simulink model "multi_level_inverter"  (Simulink 7.3)
settings: Solver=ode3  StartTime=0.0  StopTime=10  FixedStep=1e-4  RelTol=1e-3
libraries: powerlib x61, simulink x4
settings Model: Creator=Administrator  LastModifiedBy=AbdullahBaig
settings OptimizationCC: InitFltsAndDblsToZero=on
settings DebuggingCC: SaveWithParameterizedLinksMsg=none
settings RTWCC: IncludeERTFirstTime=on

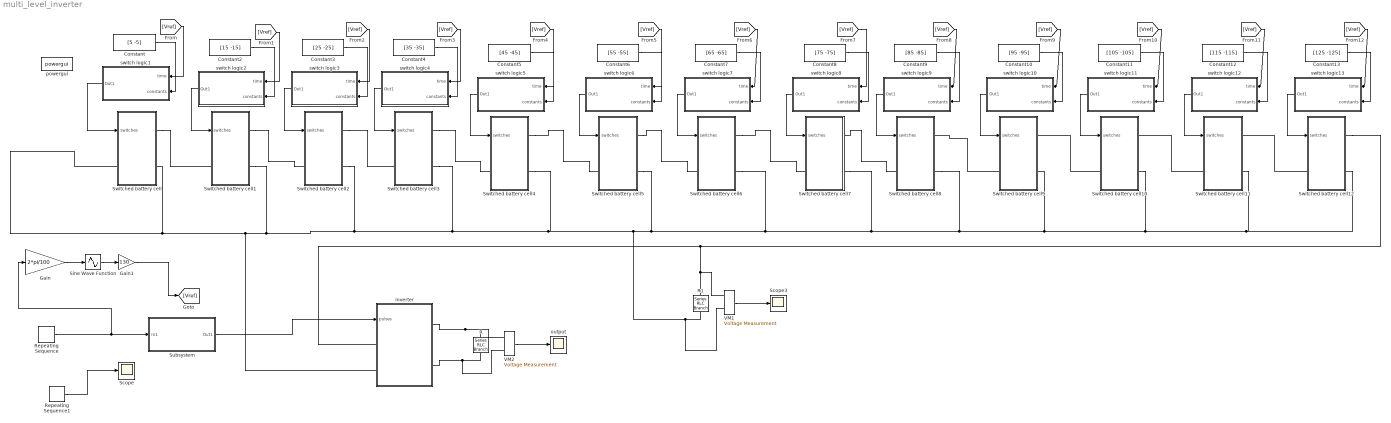
== system multi_level_inverter ==
  Constant : Constant  Value=[5 -5]  OutDataType=fixdt(1, 16)  OutScaling=2^0
  Constant10 : Constant  Value=[95 -95]  OutDataType=fixdt(1, 16)  OutScaling=2^0
  Constant11 : Constant  Value=[105 -105]  OutDataType=fixdt(1, 16)  OutScaling=2^0
  Constant12 : Constant  Value=[115 -115]  OutDataType=fixdt(1, 16)  OutScaling=2^0
  Constant13 : Constant  Value=[125 -125]  OutDataType=fixdt(1, 16)  OutScaling=2^0
  Constant2 : Constant  Value=[15 -15]  OutDataType=fixdt(1, 16)  OutScaling=2^0
  Constant3 : Constant  Value=[25 -25]  OutDataType=fixdt(1, 16)  OutScaling=2^0
  Constant4 : Constant  Value=[35 -35]  OutDataType=fixdt(1, 16)  OutScaling=2^0
  Constant5 : Constant  Value=[45 -45]  OutDataType=fixdt(1, 16)  OutScaling=2^0
  Constant6 : Constant  Value=[55 -55]  OutDataType=fixdt(1, 16)  OutScaling=2^0
  Constant7 : Constant  Value=[65 -65]  OutDataType=fixdt(1, 16)  OutScaling=2^0
  Constant8 : Constant  Value=[75 -75]  OutDataType=fixdt(1, 16)  OutScaling=2^0
  Constant9 : Constant  Value=[85 -85]  OutDataType=fixdt(1, 16)  OutScaling=2^0
  Gain : Gain  Gain=2*pi/100  ParameterDataType=fixdt(1, 16)  ParameterScaling=2^0  OutDataType=fixdt(1, 16)  OutScaling=2^0
  Gain1 : Gain  Gain=130  ParameterDataType=fixdt(1, 16)  ParameterScaling=2^0  OutDataType=fixdt(1, 16)  OutScaling=2^0
  R : powerlib/Elements/Series RLC Branch  DialogController=POWERSYS.PowerSysDialog  PhysicalDomain=powersysdomain  SubClassName=unknown  LeftPortType=p1  RightPortType=p1  LConnTagsString=__new0  RConnTagsString=__new0  BranchType=R  Resistance=500  Inductance=1.0  SetiL0=off  InitialCurrent=0  Capacitance=1.0  Setx0=off  InitialVoltage=0  Measurements=None
  R1 : powerlib/Elements/Series RLC Branch  DialogController=POWERSYS.PowerSysDialog  PhysicalDomain=powersysdomain  SubClassName=unknown  LeftPortType=p1  RightPortType=p1  LConnTagsString=__new0  RConnTagsString=__new0  BranchType=R  Resistance=500  Inductance=1.0  SetiL0=off  InitialCurrent=0  Capacitance=1.0  Setx0=off  InitialVoltage=0  Measurements=None
  Repeating Sequence : simulink/Sources/Repeating Sequence  SystemSampleTime=-1  rep_seq_t=[0 0.02]  rep_seq_y=[0 100]
  Repeating Sequence1 : simulink/Sources/Repeating Sequence  SystemSampleTime=-1  rep_seq_t=[0 0.02]  rep_seq_y=[0 100]
  Scope : Scope
      settings: SaveName=ScopeData2
  Scope3 : Scope
      settings: YMin=0  YMax=250
  Sine Wave Function : Sin  TimeSource=Use external signal  Amplitude=1  Bias=0  Frequency=1  Phase=0  Samples=10  SampleTime=0  Offset=0
  Subsystem : Subsystem
  Switched battery cell : Subsystem
  Switched battery cell1 : Subsystem
  Switched battery cell10 : Subsystem
  Switched battery cell11 : Subsystem
  Switched battery cell12 : Subsystem
  Switched battery cell2 : Subsystem
  Switched battery cell3 : Subsystem
  Switched battery cell4 : Subsystem
  Switched battery cell5 : Subsystem
  Switched battery cell6 : Subsystem
  Switched battery cell7 : Subsystem
  Switched battery cell8 : Subsystem
  Switched battery cell9 : Subsystem
  VM1 : powerlib/Measurements/Voltage Measurement  Tag=PoWeRsYsTeMmEaSuReMeNt  DialogController=POWERSYS.PowerSysDialog  SystemSampleTime=-1  PhasorSimulation=off  OutputType=Magnitude  PSBequivalent=0
  VM2 : powerlib/Measurements/Voltage Measurement  Tag=PoWeRsYsTeMmEaSuReMeNt  DialogController=POWERSYS.PowerSysDialog  SystemSampleTime=-1  PhasorSimulation=off  OutputType=Magnitude  PSBequivalent=0
  inverter : Subsystem
  output : Scope
      settings: YMin=-350  YMax=350
  powergui : powerlib/powergui  SystemSampleTime=-1  SimulationMode=Continuous  SampleTime=50e-6  frequency=60  SPID=off  DisableSnubberDevices=off  DisableRonSwitches=off  DisableVfSwitches=off  SwTol=0  Interpol=off  frequencyindice=0  echomessages=off  HookPort=off  DisplayEquations=off  FunctionMessages=off  EnableUseOfTLC=off  x0status=blocks  RestoreLinks=warning  Frange=[0:2:500]  Ylog=off  Xlog=on  ShowGrid=off  save=off  variable=ZData  ZoomFFT=on  StartTime=0.0  cycles=1  DisplayStyle=1  fundamental=60  FreqAxis=off  MaxFrequency=1000  frequencyindicesteady=1  RmsSteady=1  display=off  Ts=0  methode=off
  switch logic1 : Subsystem
  switch logic10 : Subsystem
  switch logic11 : Subsystem
  switch logic12 : Subsystem
  switch logic13 : Subsystem
  switch logic2 : Subsystem
  switch logic3 : Subsystem
  switch logic4 : Subsystem
  switch logic5 : Subsystem
  switch logic6 : Subsystem
  switch logic7 : Subsystem
  switch logic8 : Subsystem
  switch logic9 : Subsystem
  wires:
  Subsystem/1(Out1) -> inverter/1(pulses)
  VM2/1 -> output/1
  Constant/1 -> switch logic1/2(constants)
  switch logic1/1(Out1) -> Switched battery cell/1(switches)
  Gain/1 -> Sine Wave Function/1
  Sine Wave Function/1 -> Gain1/1
  switch logic2/1(Out1) -> Switched battery cell1/1(switches)
  switch logic3/1(Out1) -> Switched battery cell2/1(switches)
  switch logic4/1(Out1) -> Switched battery cell3/1(switches)
  switch logic5/1(Out1) -> Switched battery cell4/1(switches)
  Constant2/1 -> switch logic2/2(constants)
  Constant3/1 -> switch logic3/2(constants)
  Constant4/1 -> switch logic4/2(constants)
  Constant5/1 -> switch logic5/2(constants)
  switch logic6/1(Out1) -> Switched battery cell5/1(switches)
  Constant6/1 -> switch logic6/2(constants)
  switch logic7/1(Out1) -> Switched battery cell6/1(switches)
  Constant7/1 -> switch logic7/2(constants)
  switch logic8/1(Out1) -> Switched battery cell7/1(switches)
  Constant8/1 -> switch logic8/2(constants)
  switch logic9/1(Out1) -> Switched battery cell8/1(switches)
  Constant9/1 -> switch logic9/2(constants)
  Gain1/1 -> [Vref]
  [Vref] -> switch logic1/1(time)
  [Vref] -> switch logic2/1(time)
  [Vref] -> switch logic3/1(time)
  [Vref] -> switch logic4/1(time)
  [Vref] -> switch logic5/1(time)
  [Vref] -> switch logic6/1(time)
  [Vref] -> switch logic7/1(time)
  [Vref] -> switch logic8/1(time)
  [Vref] -> switch logic9/1(time)
  switch logic10/1(Out1) -> Switched battery cell9/1(switches)
  Constant10/1 -> switch logic10/2(constants)
  [Vref] -> switch logic10/1(time)
  switch logic11/1(Out1) -> Switched battery cell10/1(switches)
  Constant11/1 -> switch logic11/2(constants)
  [Vref] -> switch logic11/1(time)
  switch logic12/1(Out1) -> Switched battery cell11/1(switches)
  Constant12/1 -> switch logic12/2(constants)
  [Vref] -> switch logic12/1(time)
  switch logic13/1(Out1) -> Switched battery cell12/1(switches)
  Constant13/1 -> switch logic13/2(constants)
  [Vref] -> switch logic13/1(time)
  Repeating Sequence/1 -> Subsystem/1(In1), Gain/1
  VM1/1 -> Scope3/1
  Repeating Sequence1/1 -> Scope/1
  connections:
  inverter/RConn1 -- R/LConn1 -- VM2/LConn1
  R/RConn1 -- inverter/RConn2 -- VM2/LConn2
  R1/RConn1 -- Switched battery cell5/RConn2 -- Switched battery cell6/RConn2 -- Switched battery cell7/RConn2 -- Switched battery cell8/RConn2 -- Switched battery cell9/RConn2 -- Switched battery cell10/RConn2 -- Switched battery cell11/RConn2 -- Switched battery cell12/RConn2 -- Switched battery cell/LConn1 -- Switched battery cell/RConn2 -- inverter/LConn2 -- Switched battery cell1/RConn2 -- Switched battery cell2/RConn2 -- Switched battery cell3/RConn2 -- Switched battery cell4/RConn2 -- VM1/LConn2
  Switched battery cell1/RConn1 -- Switched battery cell2/LConn1
  Switched battery cell2/RConn1 -- Switched battery cell3/LConn1
  Switched battery cell3/RConn1 -- Switched battery cell4/LConn1
  Switched battery cell/RConn1 -- Switched battery cell1/LConn1
  Switched battery cell4/RConn1 -- Switched battery cell5/LConn1
  Switched battery cell5/RConn1 -- Switched battery cell6/LConn1
  Switched battery cell6/RConn1 -- Switched battery cell7/LConn1
  Switched battery cell7/RConn1 -- Switched battery cell8/LConn1
  Switched battery cell12/RConn1 -- inverter/LConn1 -- R1/LConn1 -- VM1/LConn1
  Switched battery cell10/LConn1 -- Switched battery cell9/RConn1
  Switched battery cell11/LConn1 -- Switched battery cell10/RConn1
  Switched battery cell12/LConn1 -- Switched battery cell11/RConn1
  Switched battery cell9/LConn1 -- Switched battery cell8/RConn1

== system multi_level_inverter/Subsystem ==
  In1 : Inport
  Compare To Constant : simulink/Logic and Bit Operations/Compare To Constant  SystemSampleTime=-1  relop=>  const=51  LogicOutDataTypeMode=uint8  ZeroCross=off
  Compare To Constant1 : simulink/Logic and Bit Operations/Compare To Constant  SystemSampleTime=-1  relop=<  const=49  LogicOutDataTypeMode=uint8  ZeroCross=off
  Mux : Mux
  Out1 : Outport
  wires:
  Compare To Constant/1 -> Mux/1, Mux/4
  In1/1 -> Compare To Constant/1, Compare To Constant1/1
  Mux/1 -> Out1/1
  Compare To Constant1/1 -> Mux/2, Mux/3

== system multi_level_inverter/Switched battery cell ==
  switches : Inport  OutDataType=fixdt(1, 16)  OutScaling=2^0
  DC Voltage Source : powerlib/Electrical Sources/DC Voltage Source  DialogController=POWERSYS.PowerSysDialog  SystemSampleTime=-1  Amplitude=24  Measurements=None
  Demux : Demux  Outputs=3
  Ideal Switch : powerlib/Power Electronics/Ideal Switch  DialogController=POWERSYS.PowerSysDialog  SystemSampleTime=-1  Ron=0.1  Lon=0  IC=0  Rs=1e5  Cs=inf  Measurements=on
  Ideal Switch1 : powerlib/Power Electronics/Ideal Switch  DialogController=POWERSYS.PowerSysDialog  SystemSampleTime=-1  Ron=0.1  Lon=0  IC=0  Rs=1e5  Cs=inf  Measurements=on
  Ideal Switch2 : powerlib/Power Electronics/Ideal Switch  DialogController=POWERSYS.PowerSysDialog  SystemSampleTime=-1  Ron=0.1  Lon=0  IC=0  Rs=1e5  Cs=inf  Measurements=on
  Conn1 : PMIOPort  Port=1  Side=Right
  Conn2 : PMIOPort  Port=2  Side=Left
  Conn4 : PMIOPort  Port=3  Side=Right
  wires:
  Demux/1 -> Ideal Switch1/1
  Demux/2 -> Ideal Switch2/1
  Demux/3 -> Ideal Switch/1
  switches/1 -> Demux/1
  connections:
  Ideal Switch1/LConn1 -- Ideal Switch2/RConn1 -- Conn2/RConn1
  DC Voltage Source/LConn1 -- Ideal Switch2/LConn1 -- Ideal Switch/RConn1
  DC Voltage Source/RConn1 -- Conn1/RConn1 -- Ideal Switch1/RConn1
  Conn4/RConn1 -- Ideal Switch/LConn1

== system multi_level_inverter/Switched battery cell1 ==
  switches : Inport  OutDataType=fixdt(1, 16)  OutScaling=2^0
  DC Voltage Source : powerlib/Electrical Sources/DC Voltage Source  DialogController=POWERSYS.PowerSysDialog  SystemSampleTime=-1  Amplitude=24  Measurements=None
  Demux : Demux  Outputs=3
  Ideal Switch : powerlib/Power Electronics/Ideal Switch  DialogController=POWERSYS.PowerSysDialog  SystemSampleTime=-1  Ron=0.1  Lon=0  IC=0  Rs=1e5  Cs=inf  Measurements=on
  Ideal Switch1 : powerlib/Power Electronics/Ideal Switch  DialogController=POWERSYS.PowerSysDialog  SystemSampleTime=-1  Ron=0.1  Lon=0  IC=0  Rs=1e5  Cs=inf  Measurements=on
  Ideal Switch2 : powerlib/Power Electronics/Ideal Switch  DialogController=POWERSYS.PowerSysDialog  SystemSampleTime=-1  Ron=0.1  Lon=0  IC=0  Rs=1e5  Cs=inf  Measurements=on
  Conn1 : PMIOPort  Port=1  Side=Right
  Conn2 : PMIOPort  Port=2  Side=Left
  Conn4 : PMIOPort  Port=3  Side=Right
  wires:
  Demux/1 -> Ideal Switch1/1
  Demux/2 -> Ideal Switch2/1
  Demux/3 -> Ideal Switch/1
  switches/1 -> Demux/1
  connections:
  Ideal Switch1/LConn1 -- Ideal Switch2/RConn1 -- Conn2/RConn1
  Ideal Switch/RConn1 -- DC Voltage Source/LConn1 -- Ideal Switch2/LConn1
  Ideal Switch1/RConn1 -- DC Voltage Source/RConn1 -- Conn1/RConn1
  Conn4/RConn1 -- Ideal Switch/LConn1

== system multi_level_inverter/Switched battery cell10 ==
  switches : Inport  OutDataType=fixdt(1, 16)  OutScaling=2^0
  DC Voltage Source : powerlib/Electrical Sources/DC Voltage Source  DialogController=POWERSYS.PowerSysDialog  SystemSampleTime=-1  Amplitude=24  Measurements=None
  Demux : Demux  Outputs=3
  Ideal Switch : powerlib/Power Electronics/Ideal Switch  DialogController=POWERSYS.PowerSysDialog  SystemSampleTime=-1  Ron=0.1  Lon=0  IC=0  Rs=1e5  Cs=inf  Measurements=on
  Ideal Switch1 : powerlib/Power Electronics/Ideal Switch  DialogController=POWERSYS.PowerSysDialog  SystemSampleTime=-1  Ron=0.1  Lon=0  IC=0  Rs=1e5  Cs=inf  Measurements=on
  Ideal Switch2 : powerlib/Power Electronics/Ideal Switch  DialogController=POWERSYS.PowerSysDialog  SystemSampleTime=-1  Ron=0.1  Lon=0  IC=0  Rs=1e5  Cs=inf  Measurements=on
  Conn1 : PMIOPort  Port=1  Side=Right
  Conn2 : PMIOPort  Port=2  Side=Left
  Conn4 : PMIOPort  Port=3  Side=Right
  wires:
  Demux/1 -> Ideal Switch1/1
  Demux/2 -> Ideal Switch2/1
  Demux/3 -> Ideal Switch/1
  switches/1 -> Demux/1
  connections:
  Ideal Switch1/LConn1 -- Ideal Switch2/RConn1 -- Conn2/RConn1
  Ideal Switch/RConn1 -- DC Voltage Source/LConn1 -- Ideal Switch2/LConn1
  Ideal Switch1/RConn1 -- DC Voltage Source/RConn1 -- Conn1/RConn1
  Conn4/RConn1 -- Ideal Switch/LConn1

== system multi_level_inverter/Switched battery cell11 ==
  switches : Inport  OutDataType=fixdt(1, 16)  OutScaling=2^0
  DC Voltage Source : powerlib/Electrical Sources/DC Voltage Source  DialogController=POWERSYS.PowerSysDialog  SystemSampleTime=-1  Amplitude=24  Measurements=None
  Demux : Demux  Outputs=3
  Ideal Switch : powerlib/Power Electronics/Ideal Switch  DialogController=POWERSYS.PowerSysDialog  SystemSampleTime=-1  Ron=0.1  Lon=0  IC=0  Rs=1e5  Cs=inf  Measurements=on
  Ideal Switch1 : powerlib/Power Electronics/Ideal Switch  DialogController=POWERSYS.PowerSysDialog  SystemSampleTime=-1  Ron=0.1  Lon=0  IC=0  Rs=1e5  Cs=inf  Measurements=on
  Ideal Switch2 : powerlib/Power Electronics/Ideal Switch  DialogController=POWERSYS.PowerSysDialog  SystemSampleTime=-1  Ron=0.1  Lon=0  IC=0  Rs=1e5  Cs=inf  Measurements=on
  Conn1 : PMIOPort  Port=1  Side=Right
  Conn2 : PMIOPort  Port=2  Side=Left
  Conn4 : PMIOPort  Port=3  Side=Right
  wires:
  Demux/1 -> Ideal Switch1/1
  Demux/2 -> Ideal Switch2/1
  Demux/3 -> Ideal Switch/1
  switches/1 -> Demux/1
  connections:
  Ideal Switch1/LConn1 -- Ideal Switch2/RConn1 -- Conn2/RConn1
  Ideal Switch/RConn1 -- DC Voltage Source/LConn1 -- Ideal Switch2/LConn1
  Ideal Switch1/RConn1 -- DC Voltage Source/RConn1 -- Conn1/RConn1
  Conn4/RConn1 -- Ideal Switch/LConn1

== system multi_level_inverter/Switched battery cell12 ==
  switches : Inport  OutDataType=fixdt(1, 16)  OutScaling=2^0
  DC Voltage Source : powerlib/Electrical Sources/DC Voltage Source  DialogController=POWERSYS.PowerSysDialog  SystemSampleTime=-1  Amplitude=24  Measurements=None
  Demux : Demux  Outputs=3
  Ideal Switch : powerlib/Power Electronics/Ideal Switch  DialogController=POWERSYS.PowerSysDialog  SystemSampleTime=-1  Ron=0.1  Lon=0  IC=0  Rs=1e5  Cs=inf  Measurements=on
  Ideal Switch1 : powerlib/Power Electronics/Ideal Switch  DialogController=POWERSYS.PowerSysDialog  SystemSampleTime=-1  Ron=0.1  Lon=0  IC=0  Rs=1e5  Cs=inf  Measurements=on
  Ideal Switch2 : powerlib/Power Electronics/Ideal Switch  DialogController=POWERSYS.PowerSysDialog  SystemSampleTime=-1  Ron=0.1  Lon=0  IC=0  Rs=1e5  Cs=inf  Measurements=on
  Conn1 : PMIOPort  Port=1  Side=Right
  Conn2 : PMIOPort  Port=2  Side=Left
  Conn4 : PMIOPort  Port=3  Side=Right
  wires:
  Demux/1 -> Ideal Switch1/1
  Demux/2 -> Ideal Switch2/1
  Demux/3 -> Ideal Switch/1
  switches/1 -> Demux/1
  connections:
  Ideal Switch1/LConn1 -- Ideal Switch2/RConn1 -- Conn2/RConn1
  Ideal Switch/RConn1 -- DC Voltage Source/LConn1 -- Ideal Switch2/LConn1
  Ideal Switch1/RConn1 -- DC Voltage Source/RConn1 -- Conn1/RConn1
  Conn4/RConn1 -- Ideal Switch/LConn1

== system multi_level_inverter/Switched battery cell2 ==
  switches : Inport  OutDataType=fixdt(1, 16)  OutScaling=2^0
  DC Voltage Source : powerlib/Electrical Sources/DC Voltage Source  DialogController=POWERSYS.PowerSysDialog  SystemSampleTime=-1  Amplitude=24  Measurements=None
  Demux : Demux  Outputs=3
  Ideal Switch : powerlib/Power Electronics/Ideal Switch  DialogController=POWERSYS.PowerSysDialog  SystemSampleTime=-1  Ron=0.1  Lon=0  IC=0  Rs=1e5  Cs=inf  Measurements=on
  Ideal Switch1 : powerlib/Power Electronics/Ideal Switch  DialogController=POWERSYS.PowerSysDialog  SystemSampleTime=-1  Ron=0.1  Lon=0  IC=0  Rs=1e5  Cs=inf  Measurements=on
  Ideal Switch2 : powerlib/Power Electronics/Ideal Switch  DialogController=POWERSYS.PowerSysDialog  SystemSampleTime=-1  Ron=0.1  Lon=0  IC=0  Rs=1e5  Cs=inf  Measurements=on
  Conn1 : PMIOPort  Port=1  Side=Right
  Conn2 : PMIOPort  Port=2  Side=Left
  Conn4 : PMIOPort  Port=3  Side=Right
  wires:
  Demux/1 -> Ideal Switch1/1
  Demux/2 -> Ideal Switch2/1
  Demux/3 -> Ideal Switch/1
  switches/1 -> Demux/1
  connections:
  Ideal Switch1/LConn1 -- Ideal Switch2/RConn1 -- Conn2/RConn1
  Ideal Switch/RConn1 -- DC Voltage Source/LConn1 -- Ideal Switch2/LConn1
  Ideal Switch1/RConn1 -- DC Voltage Source/RConn1 -- Conn1/RConn1
  Conn4/RConn1 -- Ideal Switch/LConn1

== system multi_level_inverter/Switched battery cell3 ==
  switches : Inport  OutDataType=fixdt(1, 16)  OutScaling=2^0
  DC Voltage Source : powerlib/Electrical Sources/DC Voltage Source  DialogController=POWERSYS.PowerSysDialog  SystemSampleTime=-1  Amplitude=24  Measurements=None
  Demux : Demux  Outputs=3
  Ideal Switch : powerlib/Power Electronics/Ideal Switch  DialogController=POWERSYS.PowerSysDialog  SystemSampleTime=-1  Ron=0.1  Lon=0  IC=0  Rs=1e5  Cs=inf  Measurements=on
  Ideal Switch1 : powerlib/Power Electronics/Ideal Switch  DialogController=POWERSYS.PowerSysDialog  SystemSampleTime=-1  Ron=0.1  Lon=0  IC=0  Rs=1e5  Cs=inf  Measurements=on
  Ideal Switch2 : powerlib/Power Electronics/Ideal Switch  DialogController=POWERSYS.PowerSysDialog  SystemSampleTime=-1  Ron=0.1  Lon=0  IC=0  Rs=1e5  Cs=inf  Measurements=on
  Conn1 : PMIOPort  Port=1  Side=Right
  Conn2 : PMIOPort  Port=2  Side=Left
  Conn4 : PMIOPort  Port=3  Side=Right
  wires:
  Demux/1 -> Ideal Switch1/1
  Demux/2 -> Ideal Switch2/1
  Demux/3 -> Ideal Switch/1
  switches/1 -> Demux/1
  connections:
  Ideal Switch1/LConn1 -- Ideal Switch2/RConn1 -- Conn2/RConn1
  Ideal Switch/RConn1 -- DC Voltage Source/LConn1 -- Ideal Switch2/LConn1
  Ideal Switch1/RConn1 -- DC Voltage Source/RConn1 -- Conn1/RConn1
  Conn4/RConn1 -- Ideal Switch/LConn1

== system multi_level_inverter/Switched battery cell4 ==
  switches : Inport  OutDataType=fixdt(1, 16)  OutScaling=2^0
  DC Voltage Source : powerlib/Electrical Sources/DC Voltage Source  DialogController=POWERSYS.PowerSysDialog  SystemSampleTime=-1  Amplitude=24  Measurements=None
  Demux : Demux  Outputs=3
  Ideal Switch : powerlib/Power Electronics/Ideal Switch  DialogController=POWERSYS.PowerSysDialog  SystemSampleTime=-1  Ron=0.1  Lon=0  IC=0  Rs=1e5  Cs=inf  Measurements=on
  Ideal Switch1 : powerlib/Power Electronics/Ideal Switch  DialogController=POWERSYS.PowerSysDialog  SystemSampleTime=-1  Ron=0.1  Lon=0  IC=0  Rs=1e5  Cs=inf  Measurements=on
  Ideal Switch2 : powerlib/Power Electronics/Ideal Switch  DialogController=POWERSYS.PowerSysDialog  SystemSampleTime=-1  Ron=0.1  Lon=0  IC=0  Rs=1e5  Cs=inf  Measurements=on
  Conn1 : PMIOPort  Port=1  Side=Right
  Conn2 : PMIOPort  Port=2  Side=Left
  Conn4 : PMIOPort  Port=3  Side=Right
  wires:
  Demux/1 -> Ideal Switch1/1
  Demux/2 -> Ideal Switch2/1
  Demux/3 -> Ideal Switch/1
  switches/1 -> Demux/1
  connections:
  Ideal Switch1/LConn1 -- Ideal Switch2/RConn1 -- Conn2/RConn1
  Ideal Switch/RConn1 -- DC Voltage Source/LConn1 -- Ideal Switch2/LConn1
  Ideal Switch1/RConn1 -- DC Voltage Source/RConn1 -- Conn1/RConn1
  Conn4/RConn1 -- Ideal Switch/LConn1

== system multi_level_inverter/Switched battery cell5 ==
  switches : Inport  OutDataType=fixdt(1, 16)  OutScaling=2^0
  DC Voltage Source : powerlib/Electrical Sources/DC Voltage Source  DialogController=POWERSYS.PowerSysDialog  SystemSampleTime=-1  Amplitude=24  Measurements=None
  Demux : Demux  Outputs=3
  Ideal Switch : powerlib/Power Electronics/Ideal Switch  DialogController=POWERSYS.PowerSysDialog  SystemSampleTime=-1  Ron=0.1  Lon=0  IC=0  Rs=1e5  Cs=inf  Measurements=on
  Ideal Switch1 : powerlib/Power Electronics/Ideal Switch  DialogController=POWERSYS.PowerSysDialog  SystemSampleTime=-1  Ron=0.1  Lon=0  IC=0  Rs=1e5  Cs=inf  Measurements=on
  Ideal Switch2 : powerlib/Power Electronics/Ideal Switch  DialogController=POWERSYS.PowerSysDialog  SystemSampleTime=-1  Ron=0.1  Lon=0  IC=0  Rs=1e5  Cs=inf  Measurements=on
  Conn1 : PMIOPort  Port=1  Side=Right
  Conn2 : PMIOPort  Port=2  Side=Left
  Conn4 : PMIOPort  Port=3  Side=Right
  wires:
  Demux/1 -> Ideal Switch1/1
  Demux/2 -> Ideal Switch2/1
  Demux/3 -> Ideal Switch/1
  switches/1 -> Demux/1
  connections:
  Ideal Switch1/LConn1 -- Ideal Switch2/RConn1 -- Conn2/RConn1
  Ideal Switch/RConn1 -- DC Voltage Source/LConn1 -- Ideal Switch2/LConn1
  Ideal Switch1/RConn1 -- DC Voltage Source/RConn1 -- Conn1/RConn1
  Conn4/RConn1 -- Ideal Switch/LConn1

== system multi_level_inverter/Switched battery cell6 ==
  switches : Inport  OutDataType=fixdt(1, 16)  OutScaling=2^0
  DC Voltage Source : powerlib/Electrical Sources/DC Voltage Source  DialogController=POWERSYS.PowerSysDialog  SystemSampleTime=-1  Amplitude=24  Measurements=None
  Demux : Demux  Outputs=3
  Ideal Switch : powerlib/Power Electronics/Ideal Switch  DialogController=POWERSYS.PowerSysDialog  SystemSampleTime=-1  Ron=0.1  Lon=0  IC=0  Rs=1e5  Cs=inf  Measurements=on
  Ideal Switch1 : powerlib/Power Electronics/Ideal Switch  DialogController=POWERSYS.PowerSysDialog  SystemSampleTime=-1  Ron=0.1  Lon=0  IC=0  Rs=1e5  Cs=inf  Measurements=on
  Ideal Switch2 : powerlib/Power Electronics/Ideal Switch  DialogController=POWERSYS.PowerSysDialog  SystemSampleTime=-1  Ron=0.1  Lon=0  IC=0  Rs=1e5  Cs=inf  Measurements=on
  Conn1 : PMIOPort  Port=1  Side=Right
  Conn2 : PMIOPort  Port=2  Side=Left
  Conn4 : PMIOPort  Port=3  Side=Right
  wires:
  Demux/1 -> Ideal Switch1/1
  Demux/2 -> Ideal Switch2/1
  Demux/3 -> Ideal Switch/1
  switches/1 -> Demux/1
  connections:
  Ideal Switch1/LConn1 -- Ideal Switch2/RConn1 -- Conn2/RConn1
  Ideal Switch/RConn1 -- DC Voltage Source/LConn1 -- Ideal Switch2/LConn1
  Ideal Switch1/RConn1 -- DC Voltage Source/RConn1 -- Conn1/RConn1
  Conn4/RConn1 -- Ideal Switch/LConn1

== system multi_level_inverter/Switched battery cell7 ==
  switches : Inport  OutDataType=fixdt(1, 16)  OutScaling=2^0
  DC Voltage Source : powerlib/Electrical Sources/DC Voltage Source  DialogController=POWERSYS.PowerSysDialog  SystemSampleTime=-1  Amplitude=24  Measurements=None
  Demux : Demux  Outputs=3
  Ideal Switch : powerlib/Power Electronics/Ideal Switch  DialogController=POWERSYS.PowerSysDialog  SystemSampleTime=-1  Ron=0.1  Lon=0  IC=0  Rs=1e5  Cs=inf  Measurements=on
  Ideal Switch1 : powerlib/Power Electronics/Ideal Switch  DialogController=POWERSYS.PowerSysDialog  SystemSampleTime=-1  Ron=0.1  Lon=0  IC=0  Rs=1e5  Cs=inf  Measurements=on
  Ideal Switch2 : powerlib/Power Electronics/Ideal Switch  DialogController=POWERSYS.PowerSysDialog  SystemSampleTime=-1  Ron=0.1  Lon=0  IC=0  Rs=1e5  Cs=inf  Measurements=on
  Conn1 : PMIOPort  Port=1  Side=Right
  Conn2 : PMIOPort  Port=2  Side=Left
  Conn4 : PMIOPort  Port=3  Side=Right
  wires:
  Demux/1 -> Ideal Switch1/1
  Demux/2 -> Ideal Switch2/1
  Demux/3 -> Ideal Switch/1
  switches/1 -> Demux/1
  connections:
  Ideal Switch1/LConn1 -- Ideal Switch2/RConn1 -- Conn2/RConn1
  Ideal Switch/RConn1 -- DC Voltage Source/LConn1 -- Ideal Switch2/LConn1
  Ideal Switch1/RConn1 -- DC Voltage Source/RConn1 -- Conn1/RConn1
  Conn4/RConn1 -- Ideal Switch/LConn1

== system multi_level_inverter/Switched battery cell8 ==
  switches : Inport  OutDataType=fixdt(1, 16)  OutScaling=2^0
  DC Voltage Source : powerlib/Electrical Sources/DC Voltage Source  DialogController=POWERSYS.PowerSysDialog  SystemSampleTime=-1  Amplitude=24  Measurements=None
  Demux : Demux  Outputs=3
  Ideal Switch : powerlib/Power Electronics/Ideal Switch  DialogController=POWERSYS.PowerSysDialog  SystemSampleTime=-1  Ron=0.1  Lon=0  IC=0  Rs=1e5  Cs=inf  Measurements=on
  Ideal Switch1 : powerlib/Power Electronics/Ideal Switch  DialogController=POWERSYS.PowerSysDialog  SystemSampleTime=-1  Ron=0.1  Lon=0  IC=0  Rs=1e5  Cs=inf  Measurements=on
  Ideal Switch2 : powerlib/Power Electronics/Ideal Switch  DialogController=POWERSYS.PowerSysDialog  SystemSampleTime=-1  Ron=0.1  Lon=0  IC=0  Rs=1e5  Cs=inf  Measurements=on
  Conn1 : PMIOPort  Port=1  Side=Right
  Conn2 : PMIOPort  Port=2  Side=Left
  Conn4 : PMIOPort  Port=3  Side=Right
  wires:
  Demux/1 -> Ideal Switch1/1
  Demux/2 -> Ideal Switch2/1
  Demux/3 -> Ideal Switch/1
  switches/1 -> Demux/1
  connections:
  Ideal Switch1/LConn1 -- Ideal Switch2/RConn1 -- Conn2/RConn1
  Ideal Switch/RConn1 -- DC Voltage Source/LConn1 -- Ideal Switch2/LConn1
  Ideal Switch1/RConn1 -- DC Voltage Source/RConn1 -- Conn1/RConn1
  Conn4/RConn1 -- Ideal Switch/LConn1

== system multi_level_inverter/Switched battery cell9 ==
  switches : Inport  OutDataType=fixdt(1, 16)  OutScaling=2^0
  DC Voltage Source : powerlib/Electrical Sources/DC Voltage Source  DialogController=POWERSYS.PowerSysDialog  SystemSampleTime=-1  Amplitude=24  Measurements=None
  Demux : Demux  Outputs=3
  Ideal Switch : powerlib/Power Electronics/Ideal Switch  DialogController=POWERSYS.PowerSysDialog  SystemSampleTime=-1  Ron=0.1  Lon=0  IC=0  Rs=1e5  Cs=inf  Measurements=on
  Ideal Switch1 : powerlib/Power Electronics/Ideal Switch  DialogController=POWERSYS.PowerSysDialog  SystemSampleTime=-1  Ron=0.1  Lon=0  IC=0  Rs=1e5  Cs=inf  Measurements=on
  Ideal Switch2 : powerlib/Power Electronics/Ideal Switch  DialogController=POWERSYS.PowerSysDialog  SystemSampleTime=-1  Ron=0.1  Lon=0  IC=0  Rs=1e5  Cs=inf  Measurements=on
  Conn1 : PMIOPort  Port=1  Side=Right
  Conn2 : PMIOPort  Port=2  Side=Left
  Conn4 : PMIOPort  Port=3  Side=Right
  wires:
  Demux/1 -> Ideal Switch1/1
  Demux/2 -> Ideal Switch2/1
  Demux/3 -> Ideal Switch/1
  switches/1 -> Demux/1
  connections:
  Ideal Switch1/LConn1 -- Ideal Switch2/RConn1 -- Conn2/RConn1
  Ideal Switch/RConn1 -- DC Voltage Source/LConn1 -- Ideal Switch2/LConn1
  Ideal Switch1/RConn1 -- DC Voltage Source/RConn1 -- Conn1/RConn1
  Conn4/RConn1 -- Ideal Switch/LConn1

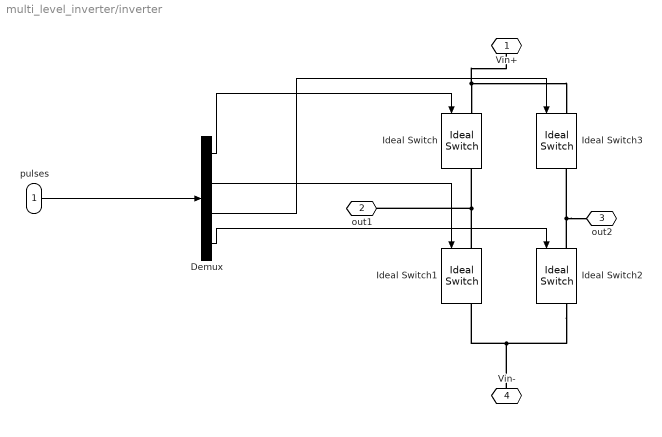
== system multi_level_inverter/inverter ==
  pulses : Inport
  Demux : Demux
  Ideal Switch{,1..3} (4 alike) : powerlib/Power Electronics/Ideal Switch  DialogController=POWERSYS.PowerSysDialog  SystemSampleTime=-1  Ron=0.001  Lon=0  IC=0  Rs=1e5  Cs=inf  Measurements=on
  Vin+ : PMIOPort  Port=1  Side=Left
  out1 : PMIOPort  Port=2  Side=Right
  out2 : PMIOPort  Port=3  Side=Right
  Vin- : PMIOPort  Port=4  Side=Left
  wires:
  Demux/1 -> Ideal Switch/1
  Demux/3 -> Ideal Switch3/1
  Demux/2 -> Ideal Switch1/1
  Demux/4 -> Ideal Switch2/1
  pulses/1 -> Demux/1
  connections:
  Vin+/RConn1 -- Ideal Switch/LConn1 -- Ideal Switch3/LConn1
  out1/RConn1 -- Ideal Switch1/LConn1 -- Ideal Switch/RConn1
  Ideal Switch2/RConn1 -- Ideal Switch1/RConn1 -- Vin-/RConn1
  out2/RConn1 -- Ideal Switch2/LConn1 -- Ideal Switch3/RConn1

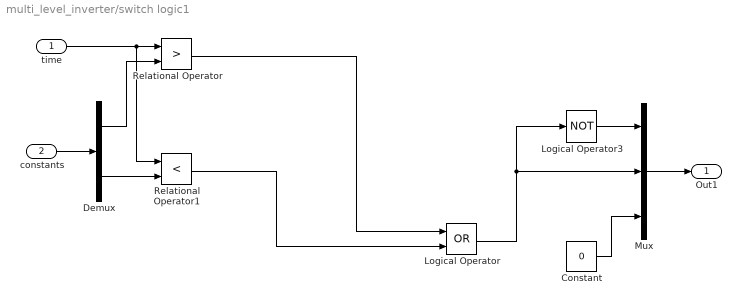
== system multi_level_inverter/switch logic1 ==
  time : Inport
  constants : Inport  Port=2
  Constant : Constant  Value=0  OutDataType=fixdt(1, 16)  OutScaling=2^0
  Demux : Demux  Outputs=2
  Logical Operator : Logic  Operator=OR  AllPortsSameDT=off  OutDataTypeMode=boolean  LogicDataType=fixdt(0, 8)  OutDataTypeStr=boolean
  Logical Operator3 : Logic  Operator=NOT  AllPortsSameDT=off  OutDataTypeMode=boolean  LogicDataType=fixdt(0, 8)  OutDataTypeStr=boolean
  Mux : Mux  Inputs=3
  Relational Operator : RelationalOperator  Operator=>  LogicOutDataTypeMode=boolean  LogicDataType=fixdt(0, 8)  OutDataTypeStr=boolean
  Relational Operator1 : RelationalOperator  Operator=<  LogicOutDataTypeMode=boolean  LogicDataType=fixdt(0, 8)  OutDataTypeStr=boolean
  Out1 : Outport
  wires:
  Mux/1 -> Out1/1
  constants/1 -> Demux/1
  Demux/1 -> Relational Operator/2
  Demux/2 -> Relational Operator1/2
  time/1 -> Relational Operator/1, Relational Operator1/1
  Constant/1 -> Mux/3
  Logical Operator/1 -> Logical Operator3/1, Mux/2
  Logical Operator3/1 -> Mux/1
  Relational Operator/1 -> Logical Operator/1
  Relational Operator1/1 -> Logical Operator/2

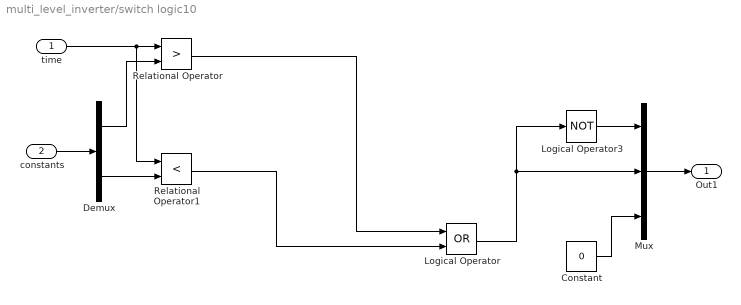
== system multi_level_inverter/switch logic10 ==
  time : Inport
  constants : Inport  Port=2
  Constant : Constant  Value=0  OutDataType=fixdt(1, 16)  OutScaling=2^0
  Demux : Demux  Outputs=2
  Logical Operator : Logic  Operator=OR  AllPortsSameDT=off  OutDataTypeMode=boolean  LogicDataType=fixdt(0, 8)  OutDataTypeStr=boolean
  Logical Operator3 : Logic  Operator=NOT  AllPortsSameDT=off  OutDataTypeMode=boolean  LogicDataType=fixdt(0, 8)  OutDataTypeStr=boolean
  Mux : Mux  Inputs=3
  Relational Operator : RelationalOperator  Operator=>  LogicOutDataTypeMode=boolean  LogicDataType=fixdt(0, 8)  OutDataTypeStr=boolean
  Relational Operator1 : RelationalOperator  Operator=<  LogicOutDataTypeMode=boolean  LogicDataType=fixdt(0, 8)  OutDataTypeStr=boolean
  Out1 : Outport
  wires:
  Mux/1 -> Out1/1
  constants/1 -> Demux/1
  Demux/1 -> Relational Operator/2
  Demux/2 -> Relational Operator1/2
  time/1 -> Relational Operator/1, Relational Operator1/1
  Constant/1 -> Mux/3
  Logical Operator/1 -> Logical Operator3/1, Mux/2
  Logical Operator3/1 -> Mux/1
  Relational Operator/1 -> Logical Operator/1
  Relational Operator1/1 -> Logical Operator/2

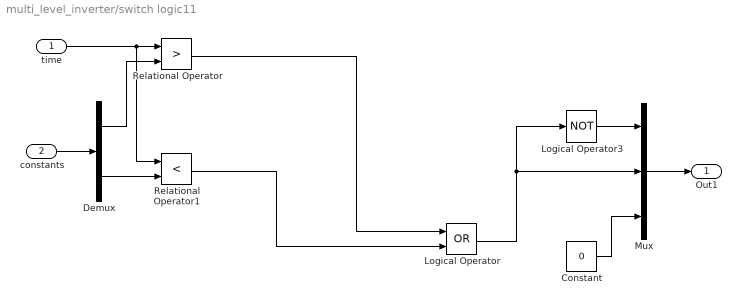
== system multi_level_inverter/switch logic11 ==
  time : Inport
  constants : Inport  Port=2
  Constant : Constant  Value=0  OutDataType=fixdt(1, 16)  OutScaling=2^0
  Demux : Demux  Outputs=2
  Logical Operator : Logic  Operator=OR  AllPortsSameDT=off  OutDataTypeMode=boolean  LogicDataType=fixdt(0, 8)  OutDataTypeStr=boolean
  Logical Operator3 : Logic  Operator=NOT  AllPortsSameDT=off  OutDataTypeMode=boolean  LogicDataType=fixdt(0, 8)  OutDataTypeStr=boolean
  Mux : Mux  Inputs=3
  Relational Operator : RelationalOperator  Operator=>  LogicOutDataTypeMode=boolean  LogicDataType=fixdt(0, 8)  OutDataTypeStr=boolean
  Relational Operator1 : RelationalOperator  Operator=<  LogicOutDataTypeMode=boolean  LogicDataType=fixdt(0, 8)  OutDataTypeStr=boolean
  Out1 : Outport
  wires:
  Mux/1 -> Out1/1
  constants/1 -> Demux/1
  Demux/1 -> Relational Operator/2
  Demux/2 -> Relational Operator1/2
  time/1 -> Relational Operator/1, Relational Operator1/1
  Constant/1 -> Mux/3
  Logical Operator/1 -> Logical Operator3/1, Mux/2
  Logical Operator3/1 -> Mux/1
  Relational Operator/1 -> Logical Operator/1
  Relational Operator1/1 -> Logical Operator/2

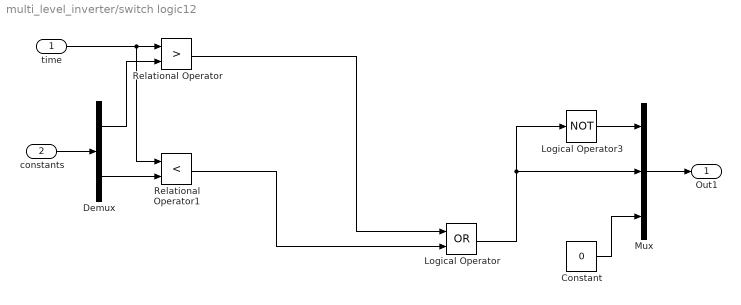
== system multi_level_inverter/switch logic12 ==
  time : Inport
  constants : Inport  Port=2
  Constant : Constant  Value=0  OutDataType=fixdt(1, 16)  OutScaling=2^0
  Demux : Demux  Outputs=2
  Logical Operator : Logic  Operator=OR  AllPortsSameDT=off  OutDataTypeMode=boolean  LogicDataType=fixdt(0, 8)  OutDataTypeStr=boolean
  Logical Operator3 : Logic  Operator=NOT  AllPortsSameDT=off  OutDataTypeMode=boolean  LogicDataType=fixdt(0, 8)  OutDataTypeStr=boolean
  Mux : Mux  Inputs=3
  Relational Operator : RelationalOperator  Operator=>  LogicOutDataTypeMode=boolean  LogicDataType=fixdt(0, 8)  OutDataTypeStr=boolean
  Relational Operator1 : RelationalOperator  Operator=<  LogicOutDataTypeMode=boolean  LogicDataType=fixdt(0, 8)  OutDataTypeStr=boolean
  Out1 : Outport
  wires:
  Mux/1 -> Out1/1
  constants/1 -> Demux/1
  Demux/1 -> Relational Operator/2
  Demux/2 -> Relational Operator1/2
  time/1 -> Relational Operator/1, Relational Operator1/1
  Constant/1 -> Mux/3
  Logical Operator/1 -> Logical Operator3/1, Mux/2
  Logical Operator3/1 -> Mux/1
  Relational Operator/1 -> Logical Operator/1
  Relational Operator1/1 -> Logical Operator/2

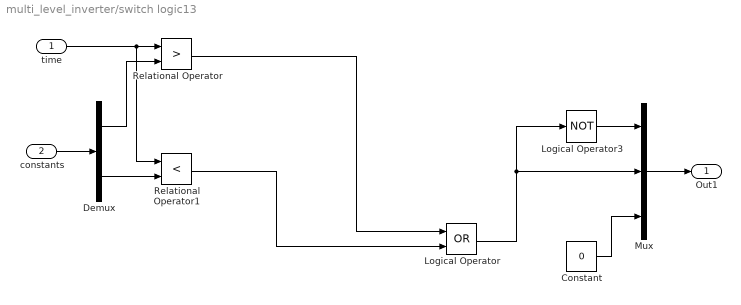
== system multi_level_inverter/switch logic13 ==
  time : Inport
  constants : Inport  Port=2
  Constant : Constant  Value=0  OutDataType=fixdt(1, 16)  OutScaling=2^0
  Demux : Demux  Outputs=2
  Logical Operator : Logic  Operator=OR  AllPortsSameDT=off  OutDataTypeMode=boolean  LogicDataType=fixdt(0, 8)  OutDataTypeStr=boolean
  Logical Operator3 : Logic  Operator=NOT  AllPortsSameDT=off  OutDataTypeMode=boolean  LogicDataType=fixdt(0, 8)  OutDataTypeStr=boolean
  Mux : Mux  Inputs=3
  Relational Operator : RelationalOperator  Operator=>  LogicOutDataTypeMode=boolean  LogicDataType=fixdt(0, 8)  OutDataTypeStr=boolean
  Relational Operator1 : RelationalOperator  Operator=<  LogicOutDataTypeMode=boolean  LogicDataType=fixdt(0, 8)  OutDataTypeStr=boolean
  Out1 : Outport
  wires:
  Mux/1 -> Out1/1
  constants/1 -> Demux/1
  Demux/1 -> Relational Operator/2
  Demux/2 -> Relational Operator1/2
  time/1 -> Relational Operator/1, Relational Operator1/1
  Constant/1 -> Mux/3
  Logical Operator/1 -> Logical Operator3/1, Mux/2
  Logical Operator3/1 -> Mux/1
  Relational Operator/1 -> Logical Operator/1
  Relational Operator1/1 -> Logical Operator/2

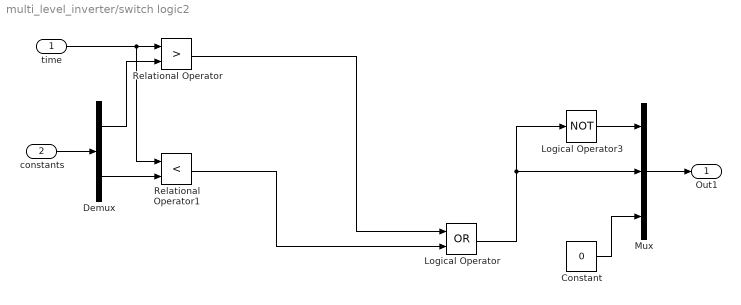
== system multi_level_inverter/switch logic2 ==
  time : Inport
  constants : Inport  Port=2
  Constant : Constant  Value=0  OutDataType=fixdt(1, 16)  OutScaling=2^0
  Demux : Demux  Outputs=2
  Logical Operator : Logic  Operator=OR  AllPortsSameDT=off  OutDataTypeMode=boolean  LogicDataType=fixdt(0, 8)  OutDataTypeStr=boolean
  Logical Operator3 : Logic  Operator=NOT  AllPortsSameDT=off  OutDataTypeMode=boolean  LogicDataType=fixdt(0, 8)  OutDataTypeStr=boolean
  Mux : Mux  Inputs=3
  Relational Operator : RelationalOperator  Operator=>  LogicOutDataTypeMode=boolean  LogicDataType=fixdt(0, 8)  OutDataTypeStr=boolean
  Relational Operator1 : RelationalOperator  Operator=<  LogicOutDataTypeMode=boolean  LogicDataType=fixdt(0, 8)  OutDataTypeStr=boolean
  Out1 : Outport
  wires:
  Mux/1 -> Out1/1
  constants/1 -> Demux/1
  Demux/1 -> Relational Operator/2
  Demux/2 -> Relational Operator1/2
  time/1 -> Relational Operator/1, Relational Operator1/1
  Constant/1 -> Mux/3
  Logical Operator/1 -> Logical Operator3/1, Mux/2
  Logical Operator3/1 -> Mux/1
  Relational Operator/1 -> Logical Operator/1
  Relational Operator1/1 -> Logical Operator/2

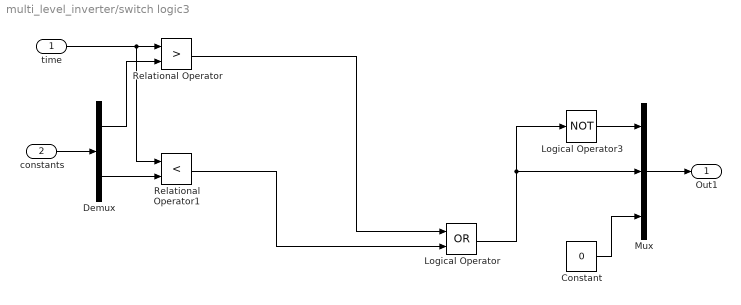
== system multi_level_inverter/switch logic3 ==
  time : Inport
  constants : Inport  Port=2
  Constant : Constant  Value=0  OutDataType=fixdt(1, 16)  OutScaling=2^0
  Demux : Demux  Outputs=2
  Logical Operator : Logic  Operator=OR  AllPortsSameDT=off  OutDataTypeMode=boolean  LogicDataType=fixdt(0, 8)  OutDataTypeStr=boolean
  Logical Operator3 : Logic  Operator=NOT  AllPortsSameDT=off  OutDataTypeMode=boolean  LogicDataType=fixdt(0, 8)  OutDataTypeStr=boolean
  Mux : Mux  Inputs=3
  Relational Operator : RelationalOperator  Operator=>  LogicOutDataTypeMode=boolean  LogicDataType=fixdt(0, 8)  OutDataTypeStr=boolean
  Relational Operator1 : RelationalOperator  Operator=<  LogicOutDataTypeMode=boolean  LogicDataType=fixdt(0, 8)  OutDataTypeStr=boolean
  Out1 : Outport
  wires:
  Mux/1 -> Out1/1
  constants/1 -> Demux/1
  Demux/1 -> Relational Operator/2
  Demux/2 -> Relational Operator1/2
  time/1 -> Relational Operator/1, Relational Operator1/1
  Constant/1 -> Mux/3
  Logical Operator/1 -> Logical Operator3/1, Mux/2
  Logical Operator3/1 -> Mux/1
  Relational Operator/1 -> Logical Operator/1
  Relational Operator1/1 -> Logical Operator/2

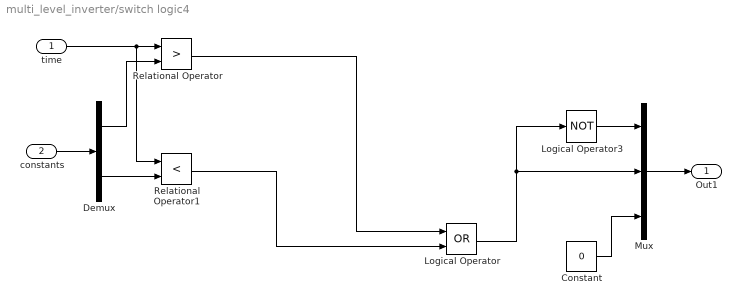
== system multi_level_inverter/switch logic4 ==
  time : Inport
  constants : Inport  Port=2
  Constant : Constant  Value=0  OutDataType=fixdt(1, 16)  OutScaling=2^0
  Demux : Demux  Outputs=2
  Logical Operator : Logic  Operator=OR  AllPortsSameDT=off  OutDataTypeMode=boolean  LogicDataType=fixdt(0, 8)  OutDataTypeStr=boolean
  Logical Operator3 : Logic  Operator=NOT  AllPortsSameDT=off  OutDataTypeMode=boolean  LogicDataType=fixdt(0, 8)  OutDataTypeStr=boolean
  Mux : Mux  Inputs=3
  Relational Operator : RelationalOperator  Operator=>  LogicOutDataTypeMode=boolean  LogicDataType=fixdt(0, 8)  OutDataTypeStr=boolean
  Relational Operator1 : RelationalOperator  Operator=<  LogicOutDataTypeMode=boolean  LogicDataType=fixdt(0, 8)  OutDataTypeStr=boolean
  Out1 : Outport
  wires:
  Mux/1 -> Out1/1
  constants/1 -> Demux/1
  Demux/1 -> Relational Operator/2
  Demux/2 -> Relational Operator1/2
  time/1 -> Relational Operator/1, Relational Operator1/1
  Constant/1 -> Mux/3
  Logical Operator/1 -> Logical Operator3/1, Mux/2
  Logical Operator3/1 -> Mux/1
  Relational Operator/1 -> Logical Operator/1
  Relational Operator1/1 -> Logical Operator/2

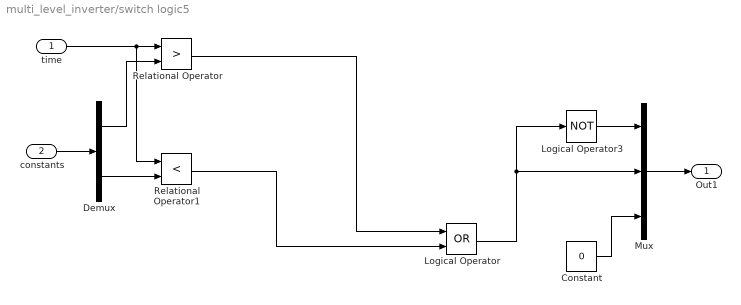
== system multi_level_inverter/switch logic5 ==
  time : Inport
  constants : Inport  Port=2
  Constant : Constant  Value=0  OutDataType=fixdt(1, 16)  OutScaling=2^0
  Demux : Demux  Outputs=2
  Logical Operator : Logic  Operator=OR  AllPortsSameDT=off  OutDataTypeMode=boolean  LogicDataType=fixdt(0, 8)  OutDataTypeStr=boolean
  Logical Operator3 : Logic  Operator=NOT  AllPortsSameDT=off  OutDataTypeMode=boolean  LogicDataType=fixdt(0, 8)  OutDataTypeStr=boolean
  Mux : Mux  Inputs=3
  Relational Operator : RelationalOperator  Operator=>  LogicOutDataTypeMode=boolean  LogicDataType=fixdt(0, 8)  OutDataTypeStr=boolean
  Relational Operator1 : RelationalOperator  Operator=<  LogicOutDataTypeMode=boolean  LogicDataType=fixdt(0, 8)  OutDataTypeStr=boolean
  Out1 : Outport
  wires:
  Mux/1 -> Out1/1
  constants/1 -> Demux/1
  Demux/1 -> Relational Operator/2
  Demux/2 -> Relational Operator1/2
  time/1 -> Relational Operator/1, Relational Operator1/1
  Constant/1 -> Mux/3
  Logical Operator/1 -> Logical Operator3/1, Mux/2
  Logical Operator3/1 -> Mux/1
  Relational Operator/1 -> Logical Operator/1
  Relational Operator1/1 -> Logical Operator/2

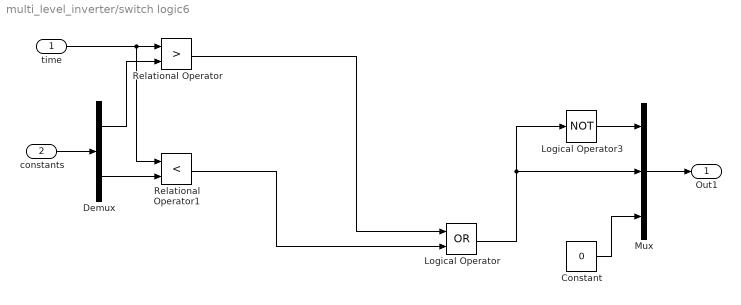
== system multi_level_inverter/switch logic6 ==
  time : Inport
  constants : Inport  Port=2
  Constant : Constant  Value=0  OutDataType=fixdt(1, 16)  OutScaling=2^0
  Demux : Demux  Outputs=2
  Logical Operator : Logic  Operator=OR  AllPortsSameDT=off  OutDataTypeMode=boolean  LogicDataType=fixdt(0, 8)  OutDataTypeStr=boolean
  Logical Operator3 : Logic  Operator=NOT  AllPortsSameDT=off  OutDataTypeMode=boolean  LogicDataType=fixdt(0, 8)  OutDataTypeStr=boolean
  Mux : Mux  Inputs=3
  Relational Operator : RelationalOperator  Operator=>  LogicOutDataTypeMode=boolean  LogicDataType=fixdt(0, 8)  OutDataTypeStr=boolean
  Relational Operator1 : RelationalOperator  Operator=<  LogicOutDataTypeMode=boolean  LogicDataType=fixdt(0, 8)  OutDataTypeStr=boolean
  Out1 : Outport
  wires:
  Mux/1 -> Out1/1
  constants/1 -> Demux/1
  Demux/1 -> Relational Operator/2
  Demux/2 -> Relational Operator1/2
  time/1 -> Relational Operator/1, Relational Operator1/1
  Constant/1 -> Mux/3
  Logical Operator/1 -> Logical Operator3/1, Mux/2
  Logical Operator3/1 -> Mux/1
  Relational Operator/1 -> Logical Operator/1
  Relational Operator1/1 -> Logical Operator/2

== system multi_level_inverter/switch logic7 ==
  time : Inport
  constants : Inport  Port=2
  Constant : Constant  Value=0  OutDataType=fixdt(1, 16)  OutScaling=2^0
  Demux : Demux  Outputs=2
  Logical Operator : Logic  Operator=OR  AllPortsSameDT=off  OutDataTypeMode=boolean  LogicDataType=fixdt(0, 8)  OutDataTypeStr=boolean
  Logical Operator3 : Logic  Operator=NOT  AllPortsSameDT=off  OutDataTypeMode=boolean  LogicDataType=fixdt(0, 8)  OutDataTypeStr=boolean
  Mux : Mux  Inputs=3
  Relational Operator : RelationalOperator  Operator=>  LogicOutDataTypeMode=boolean  LogicDataType=fixdt(0, 8)  OutDataTypeStr=boolean
  Relational Operator1 : RelationalOperator  Operator=<  LogicOutDataTypeMode=boolean  LogicDataType=fixdt(0, 8)  OutDataTypeStr=boolean
  Out1 : Outport
  wires:
  Mux/1 -> Out1/1
  constants/1 -> Demux/1
  Demux/1 -> Relational Operator/2
  Demux/2 -> Relational Operator1/2
  time/1 -> Relational Operator/1, Relational Operator1/1
  Constant/1 -> Mux/3
  Logical Operator/1 -> Logical Operator3/1, Mux/2
  Logical Operator3/1 -> Mux/1
  Relational Operator/1 -> Logical Operator/1
  Relational Operator1/1 -> Logical Operator/2

== system multi_level_inverter/switch logic8 ==
  time : Inport
  constants : Inport  Port=2
  Constant : Constant  Value=0  OutDataType=fixdt(1, 16)  OutScaling=2^0
  Demux : Demux  Outputs=2
  Logical Operator : Logic  Operator=OR  AllPortsSameDT=off  OutDataTypeMode=boolean  LogicDataType=fixdt(0, 8)  OutDataTypeStr=boolean
  Logical Operator3 : Logic  Operator=NOT  AllPortsSameDT=off  OutDataTypeMode=boolean  LogicDataType=fixdt(0, 8)  OutDataTypeStr=boolean
  Mux : Mux  Inputs=3
  Relational Operator : RelationalOperator  Operator=>  LogicOutDataTypeMode=boolean  LogicDataType=fixdt(0, 8)  OutDataTypeStr=boolean
  Relational Operator1 : RelationalOperator  Operator=<  LogicOutDataTypeMode=boolean  LogicDataType=fixdt(0, 8)  OutDataTypeStr=boolean
  Out1 : Outport
  wires:
  Mux/1 -> Out1/1
  constants/1 -> Demux/1
  Demux/1 -> Relational Operator/2
  Demux/2 -> Relational Operator1/2
  time/1 -> Relational Operator/1, Relational Operator1/1
  Constant/1 -> Mux/3
  Logical Operator/1 -> Logical Operator3/1, Mux/2
  Logical Operator3/1 -> Mux/1
  Relational Operator/1 -> Logical Operator/1
  Relational Operator1/1 -> Logical Operator/2

== system multi_level_inverter/switch logic9 ==
  time : Inport
  constants : Inport  Port=2
  Constant : Constant  Value=0  OutDataType=fixdt(1, 16)  OutScaling=2^0
  Demux : Demux  Outputs=2
  Logical Operator : Logic  Operator=OR  AllPortsSameDT=off  OutDataTypeMode=boolean  LogicDataType=fixdt(0, 8)  OutDataTypeStr=boolean
  Logical Operator3 : Logic  Operator=NOT  AllPortsSameDT=off  OutDataTypeMode=boolean  LogicDataType=fixdt(0, 8)  OutDataTypeStr=boolean
  Mux : Mux  Inputs=3
  Relational Operator : RelationalOperator  Operator=>  LogicOutDataTypeMode=boolean  LogicDataType=fixdt(0, 8)  OutDataTypeStr=boolean
  Relational Operator1 : RelationalOperator  Operator=<  LogicOutDataTypeMode=boolean  LogicDataType=fixdt(0, 8)  OutDataTypeStr=boolean
  Out1 : Outport
  wires:
  Mux/1 -> Out1/1
  constants/1 -> Demux/1
  Demux/1 -> Relational Operator/2
  Demux/2 -> Relational Operator1/2
  time/1 -> Relational Operator/1, Relational Operator1/1
  Constant/1 -> Mux/3
  Logical Operator/1 -> Logical Operator3/1, Mux/2
  Logical Operator3/1 -> Mux/1
  Relational Operator/1 -> Logical Operator/1
  Relational Operator1/1 -> Logical Operator/2
